simulink model "Sensor"  (R2023b)
settings: Solver=VariableStepAuto  StartTime=0.0  StopTime=10.0  RelTol=1e-3
values from neighbouring files (symbols this model uses):
  a_E_S = 1.495978707e8    (= 149597870.7)    [Sensors.m]
  am2 = 1    [Sensors.m]
  dP = zeros(lenn,lenm)    [Sensors.m]
  Error_horizon = 1.5*pi/180    (= 0.0261799387799)    [Sensors.m]
  Error_mag_HYST = (0.6*60e-6)    (= 3.6e-05)    [Sensors.m]
  Error_mag_ORTHO = deg2rad(0.5)    [Sensors.m]
  Error_sun = 0.5*pi/180    (= 0.00872664625997)    [Sensors.m]
  gnm = Snm.*gnm    [Sensors.m]
  hnm = Snm.*hnm    [Sensors.m]
  i_E = deg2rad(23.45)    [Sensors.m]
  n_E = 2*pi/(365*24*3600)    (= 1.99238499086e-07)    [Sensors.m]
  P = zeros(lenn,lenm)    [Sensors.m]
  R_E = 6371e3    (= 6371000)    [Sensors.m]
  T = 1    [Sensors.m]    (also in sim_with_sensors.m = 2*pi/n)
  w_E = 2*pi/(23*3600+56*60+47)    (= 7.28848621014e-05)    [Sensors.m]
libraries: dspsrcs4 x18, vrlib x2, matrix_library x1, simulink_extras x1
settings Model: Creator=TamimHR  LastModifiedBy=TamimHR

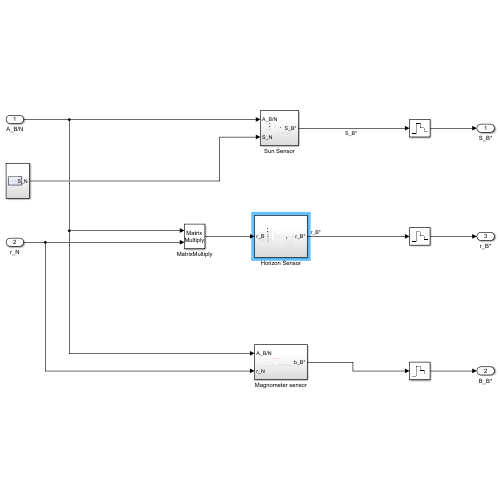
[thumbnail: Simulink's stored preview of the top-level diagram]
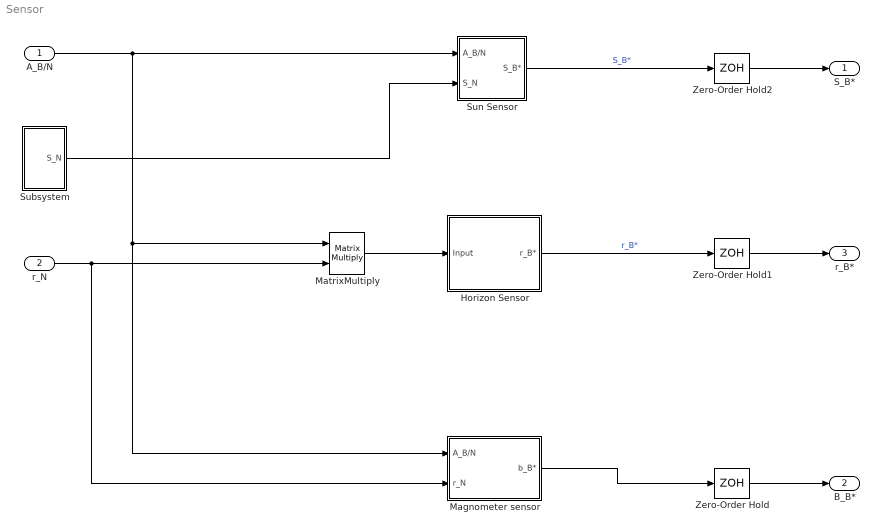
== system Sensor ==
  A_B/N : Inport
  r_N : Inport  Port=2
  Horizon Sensor : Subsystem
  Magnometer sensor : Subsystem
  MatrixMultiply : Product  Multiplication=Matrix(*)
  Subsystem : Subsystem
  Sun Sensor : Subsystem
  Zero-Order Hold : ZeroOrderHold  SampleTime=T
  Zero-Order Hold1 : ZeroOrderHold  SampleTime=T
  Zero-Order Hold2 : ZeroOrderHold  SampleTime=T
  S_B* : Outport
  B_B* : Outport  Port=2
  r_B* : Outport  Port=3
  wires:
  Zero-Order Hold2/1 -> S_B*/1
  A_B/N/1 -> Magnometer sensor/1(A_B/N), MatrixMultiply/1, Sun Sensor/1(A_B/N)
  Sun Sensor/1(S_B*) -> Zero-Order Hold2/1  "S_B*"
  Subsystem/1(S_N) -> Sun Sensor/2(S_N)
  Zero-Order Hold1/1 -> r_B*/1
  Horizon Sensor/1(r_B*) -> Zero-Order Hold1/1  "r_B*"
  r_N/1 -> Magnometer sensor/2(r_N), MatrixMultiply/2
  MatrixMultiply/1 -> Horizon Sensor/1(Input)
  Magnometer sensor/1(b_B*) -> Zero-Order Hold/1
  Zero-Order Hold/1 -> B_B*/1

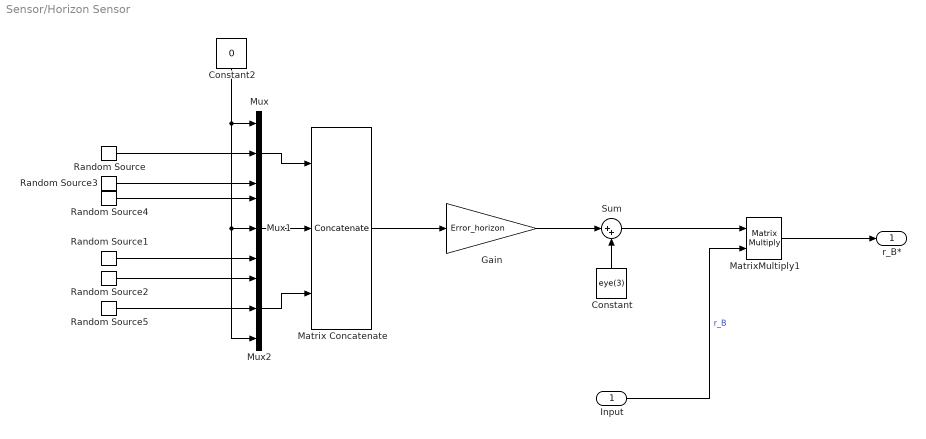
== system Sensor/Horizon Sensor ==
  Input : Inport
  Constant : Constant  Value=eye(3)
  Constant2 : Constant  Value=0
  Gain : Gain  Gain=Error_horizon
  Matrix Concatenate : Concatenate  NumInputs=3  Mode=Multidimensional array  ConcatenateDimension=2
  MatrixMultiply1 : Product  Multiplication=Matrix(*)
  Mux : Mux  Inputs=3
  Mux1 : Mux  Inputs=3
  Mux2 : Mux  Inputs=3
  Random Source : dspsrcs4/Random Source  SrcType=Uniform  NormMethod=Ziggurat  CltLength=12  MinVal=0  MaxVal=1  MeanVal=0  VarVal=1  RepMode=Not repeatable  rawSeed=1  IsInherit=off  SampMode=Discrete  SampTime=1  SampFrame=1  DataType=Double  OutComplex=Real  OutputFrames=off
  Random Source1 : dspsrcs4/Random Source  SrcType=Uniform  NormMethod=Ziggurat  CltLength=12  MinVal=0  MaxVal=1  MeanVal=0  VarVal=1  RepMode=Not repeatable  rawSeed=1  IsInherit=off  SampMode=Discrete  SampTime=1  SampFrame=1  DataType=Double  OutComplex=Real  OutputFrames=off
  Random Source2 : dspsrcs4/Random Source  SrcType=Uniform  NormMethod=Ziggurat  CltLength=12  MinVal=0  MaxVal=1  MeanVal=0  VarVal=1  RepMode=Not repeatable  rawSeed=1  IsInherit=off  SampMode=Discrete  SampTime=1  SampFrame=1  DataType=Double  OutComplex=Real  OutputFrames=off
  Random Source3 : dspsrcs4/Random Source  SrcType=Uniform  NormMethod=Ziggurat  CltLength=12  MinVal=-1  MaxVal=0  MeanVal=0  VarVal=1  RepMode=Not repeatable  rawSeed=1  IsInherit=off  SampMode=Discrete  SampTime=1  SampFrame=1  DataType=Double  OutComplex=Real  OutputFrames=off
  Random Source4 : dspsrcs4/Random Source  SrcType=Uniform  NormMethod=Ziggurat  CltLength=12  MinVal=-1  MaxVal=0  MeanVal=0  VarVal=1  RepMode=Not repeatable  rawSeed=1  IsInherit=off  SampMode=Discrete  SampTime=1  SampFrame=1  DataType=Double  OutComplex=Real  OutputFrames=off
  Random Source5 : dspsrcs4/Random Source  SrcType=Uniform  NormMethod=Ziggurat  CltLength=12  MinVal=-1  MaxVal=0  MeanVal=0  VarVal=1  RepMode=Not repeatable  rawSeed=1  IsInherit=off  SampMode=Discrete  SampTime=1  SampFrame=1  DataType=Double  OutComplex=Real  OutputFrames=off
  Sum : Sum  Inputs=|++
  r_B* : Outport
  wires:
  MatrixMultiply1/1 -> r_B*/1
  Constant2/1 -> Mux/1, Mux1/2, Mux2/3
  Matrix Concatenate/1 -> Gain/1
  Random Source/1 -> Mux/2
  Random Source1/1 -> Mux1/3
  Random Source2/1 -> Mux2/1
  Random Source3/1 -> Mux/3
  Random Source4/1 -> Mux1/1
  Random Source5/1 -> Mux2/2
  Gain/1 -> Sum/1
  Constant/1 -> Sum/2
  Sum/1 -> MatrixMultiply1/1
  Input/1 -> MatrixMultiply1/2  "r_B"
  Mux/1 -> Matrix Concatenate/1
  Mux1/1 -> Matrix Concatenate/2
  Mux2/1 -> Matrix Concatenate/3

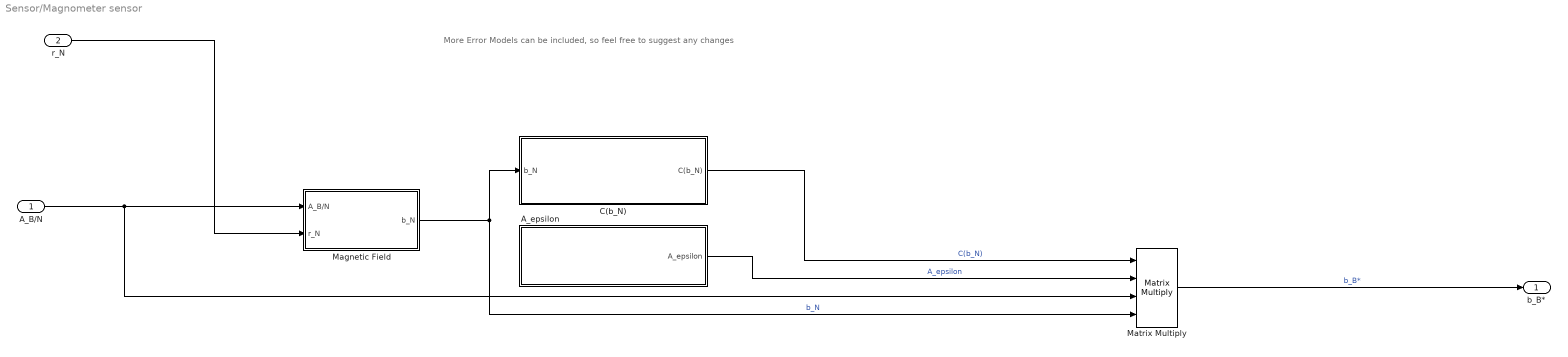
== system Sensor/Magnometer sensor ==
  note: More Error Models can be included, so feel free to suggest any changes
  A_B/N : Inport
  r_N : Inport  Port=2
  A_epsilon : Subsystem
  C(b_N) : Subsystem
  Magnetic Field : Subsystem
  Matrix Multiply : Product  Inputs=4  Multiplication=Matrix(*)
  b_B* : Outport
  wires:
  Matrix Multiply/1 -> b_B*/1  "b_B*"
  A_B/N/1 -> Matrix Multiply/3, Magnetic Field/1(A_B/N)
  Magnetic Field/1(b_N) -> Matrix Multiply/4, C(b_N)/1(b_N)  "b_N"
  A_epsilon/1(A_epsilon) -> Matrix Multiply/2  "A_epsilon"
  C(b_N)/1(C(b_N)) -> Matrix Multiply/1  "C(b_N)"
  r_N/1 -> Magnetic Field/2(r_N)

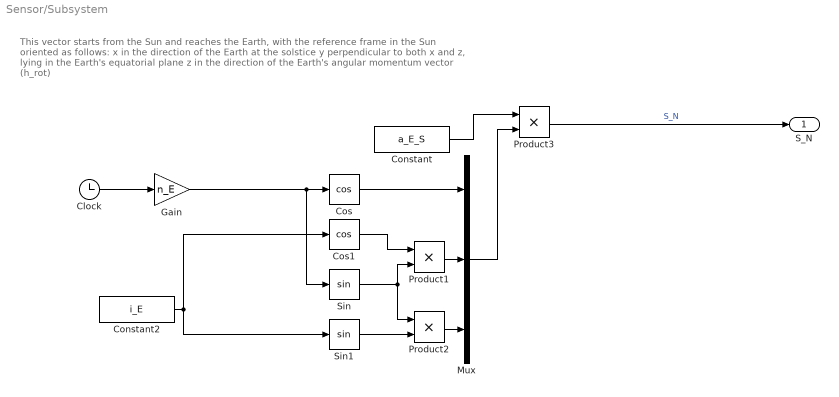
== system Sensor/Subsystem ==
  note: This vector starts from the Sun and reaches the Earth, with the reference frame in the Sun oriented as follows:
      | x in the direction of the Earth at the solstice
      | y perpendicular to both x and z, lying in the Earth's equatorial plane
      | z in the direction of the Earth's angular momentum vector (h_rot)
  Clock : Clock
  Constant : Constant  Value=a_E_S
  Constant2 : Constant  Value=i_E
  Cos : Trigonometry  Operator=cos
  Cos1 : Trigonometry  Operator=cos
  Gain : Gain  Gain=n_E
  Mux : Mux  Inputs=3
  Product1 : Product
  Product2 : Product
  Product3 : Product
  Sin : Trigonometry
  Sin1 : Trigonometry
  S_N : Outport
  wires:
  Gain/1 -> Sin/1, Cos/1
  Clock/1 -> Gain/1
  Mux/1 -> Product3/2
  Sin1/1 -> Product2/2
  Constant/1 -> Product3/1
  Constant2/1 -> Sin1/1, Cos1/1
  Product2/1 -> Mux/3
  Sin/1 -> Product1/2, Product2/1
  Cos1/1 -> Product1/1
  Cos/1 -> Mux/1
  Product1/1 -> Mux/2
  Product3/1 -> S_N/1  "S_N"

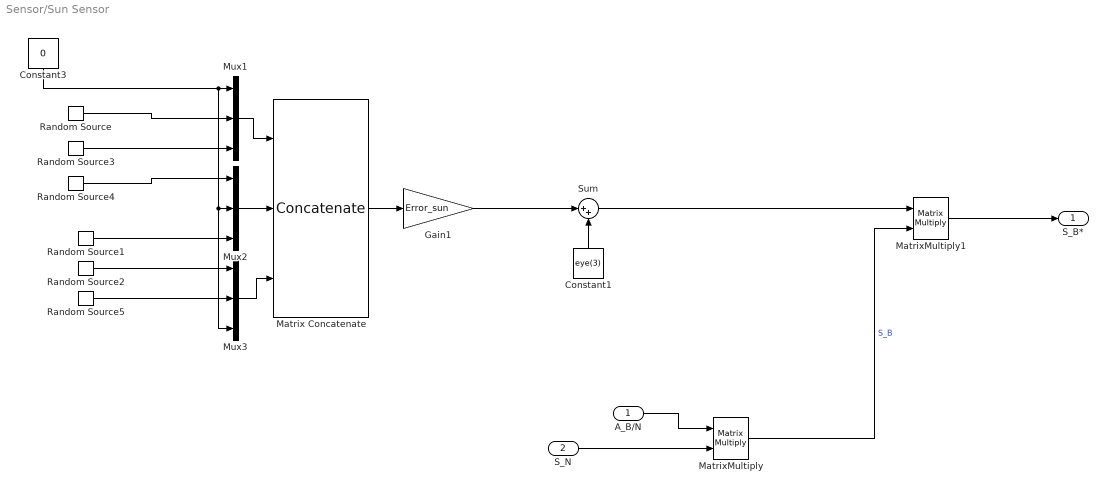
== system Sensor/Sun Sensor ==
  A_B/N : Inport
  S_N : Inport  Port=2
  Constant1 : Constant  Value=eye(3)
  Constant3 : Constant  Value=0
  Gain1 : Gain  Gain=Error_sun
  Matrix Concatenate : Concatenate  NumInputs=3  Mode=Multidimensional array  ConcatenateDimension=2
  MatrixMultiply : Product  Multiplication=Matrix(*)
  MatrixMultiply1 : Product  Multiplication=Matrix(*)
  Mux1 : Mux  Inputs=3
  Mux2 : Mux  Inputs=3
  Mux3 : Mux  Inputs=3
  Random Source : dspsrcs4/Random Source  SrcType=Uniform  NormMethod=Ziggurat  CltLength=12  MinVal=0  MaxVal=1  MeanVal=0  VarVal=1  RepMode=Not repeatable  rawSeed=1  IsInherit=off  SampMode=Discrete  SampTime=1  SampFrame=1  DataType=Double  OutComplex=Real  OutputFrames=off
  Random Source1 : dspsrcs4/Random Source  SrcType=Uniform  NormMethod=Ziggurat  CltLength=12  MinVal=0  MaxVal=1  MeanVal=0  VarVal=1  RepMode=Not repeatable  rawSeed=1  IsInherit=off  SampMode=Discrete  SampTime=1  SampFrame=1  DataType=Double  OutComplex=Real  OutputFrames=off
  Random Source2 : dspsrcs4/Random Source  SrcType=Uniform  NormMethod=Ziggurat  CltLength=12  MinVal=0  MaxVal=1  MeanVal=0  VarVal=1  RepMode=Not repeatable  rawSeed=1  IsInherit=off  SampMode=Discrete  SampTime=1  SampFrame=1  DataType=Double  OutComplex=Real  OutputFrames=off
  Random Source3 : dspsrcs4/Random Source  SrcType=Uniform  NormMethod=Ziggurat  CltLength=12  MinVal=-1  MaxVal=0  MeanVal=0  VarVal=1  RepMode=Not repeatable  rawSeed=1  IsInherit=off  SampMode=Discrete  SampTime=1  SampFrame=1  DataType=Double  OutComplex=Real  OutputFrames=off
  Random Source4 : dspsrcs4/Random Source  SrcType=Uniform  NormMethod=Ziggurat  CltLength=12  MinVal=-1  MaxVal=0  MeanVal=0  VarVal=1  RepMode=Not repeatable  rawSeed=1  IsInherit=off  SampMode=Discrete  SampTime=1  SampFrame=1  DataType=Double  OutComplex=Real  OutputFrames=off
  Random Source5 : dspsrcs4/Random Source  SrcType=Uniform  NormMethod=Ziggurat  CltLength=12  MinVal=-1  MaxVal=0  MeanVal=0  VarVal=1  RepMode=Not repeatable  rawSeed=1  IsInherit=off  SampMode=Discrete  SampTime=1  SampFrame=1  DataType=Double  OutComplex=Real  OutputFrames=off
  Sum : Sum  Inputs=|++
  S_B* : Outport
  wires:
  Constant3/1 -> Mux2/2, Mux3/3, Mux1/1
  Sum/1 -> MatrixMultiply1/1
  Random Source2/1 -> Mux3/1
  Random Source4/1 -> Mux2/1
  Constant1/1 -> Sum/2
  MatrixMultiply/1 -> MatrixMultiply1/2  "S_B"
  A_B/N/1 -> MatrixMultiply/1
  MatrixMultiply1/1 -> S_B*/1
  Mux3/1 -> Matrix Concatenate/3
  Mux2/1 -> Matrix Concatenate/2
  Mux1/1 -> Matrix Concatenate/1
  Random Source5/1 -> Mux3/2
  Random Source/1 -> Mux1/2
  Gain1/1 -> Sum/1
  Random Source1/1 -> Mux2/3
  Random Source3/1 -> Mux1/3
  Matrix Concatenate/1 -> Gain1/1
  S_N/1 -> MatrixMultiply/2

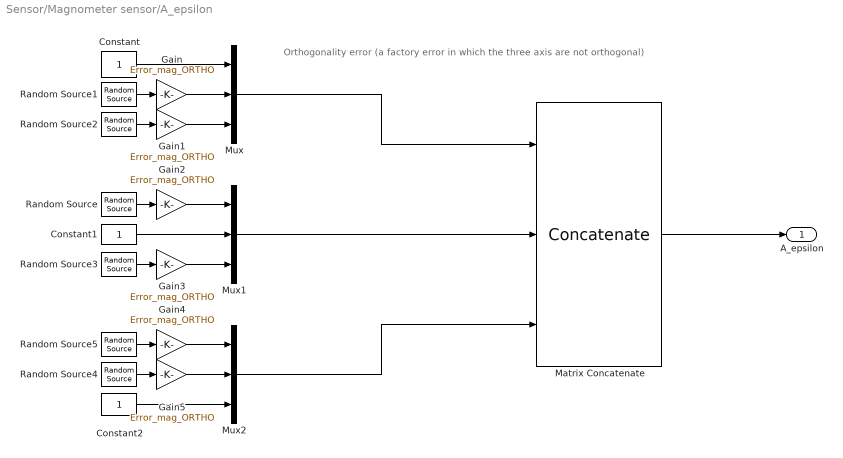
== system Sensor/Magnometer sensor/A_epsilon ==
  note: Orthogonality error (a factory error in which the three axis are not orthogonal)
  Constant : Constant
  Constant1 : Constant
  Constant2 : Constant
  Gain{,1..5} (6 alike) : Gain  Gain=Error_mag_ORTHO
  Matrix Concatenate : Concatenate  NumInputs=3  Mode=Multidimensional array  ConcatenateDimension=2
  Mux : Mux  Inputs=3
  Mux1 : Mux  Inputs=3
  Mux2 : Mux  Inputs=3
  Random Source{,1..5} (6 alike) : dspsrcs4/Random Source  SrcType=Uniform  NormMethod=Ziggurat  CltLength=12  MinVal=-1  MaxVal=1  MeanVal=0  VarVal=25  RepMode=Not repeatable  rawSeed=1  IsInherit=off  SampMode=Continuous  SampTime=1  SampFrame=1  DataType=Double  OutComplex=Real  OutputFrames=off
  A_epsilon : Outport
  wires:
  Random Source4/1 -> Gain5/1
  Constant/1 -> Mux/1
  Mux/1 -> Matrix Concatenate/1
  Random Source1/1 -> Gain/1
  Random Source/1 -> Gain2/1
  Mux1/1 -> Matrix Concatenate/2
  Random Source2/1 -> Gain1/1
  Random Source3/1 -> Gain3/1
  Random Source5/1 -> Gain4/1
  Mux2/1 -> Matrix Concatenate/3
  Matrix Concatenate/1 -> A_epsilon/1
  Gain/1 -> Mux/2
  Gain1/1 -> Mux/3
  Gain2/1 -> Mux1/1
  Gain3/1 -> Mux1/3
  Gain4/1 -> Mux2/1
  Gain5/1 -> Mux2/2
  Constant1/1 -> Mux1/2
  Constant2/1 -> Mux2/3

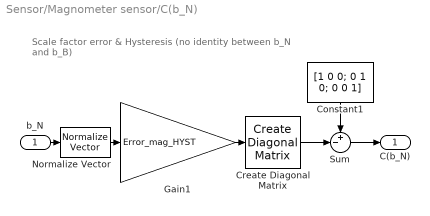
== system Sensor/Magnometer sensor/C(b_N) ==
  note: Scale factor error & Hysteresis (no identity between b_N and b_B)
  b_N : Inport
  Constant1 : Constant  Value=[1 0 0; 0 1 0; 0 0 1]
  Create Diagonal Matrix : matrix_library/Create Diagonal Matrix
      settings: LibrarySourceBlock=|
      | simulink/Matrix
      | Operations/Create Diagonal
      | Matrix
  Gain1 : Gain  Gain=Error_mag_HYST
  Normalize Vector : vrlib/Utilities/Normalize Vector  maxzero=0
  Sum : Sum  Inputs=+-|
  C(b_N) : Outport
  wires:
  Normalize Vector/1 -> Gain1/1
  Gain1/1 -> Create Diagonal Matrix/1
  Constant1/1 -> Sum/1
  Sum/1 -> C(b_N)/1
  b_N/1 -> Normalize Vector/1
  Create Diagonal Matrix/1 -> Sum/2

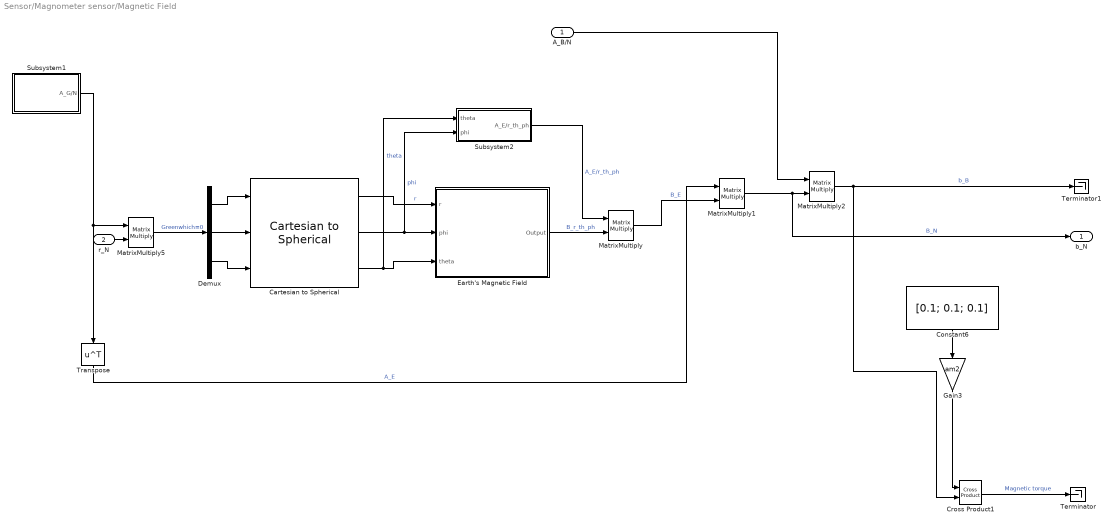
== system Sensor/Magnometer sensor/Magnetic Field ==
  A_B/N : Inport
  r_N : Inport  Port=2
  Cartesian to Spherical : simulink_extras/Transformations/Cartesian to Spherical
  Constant6 : Constant  Value=[0.1; 0.1; 0.1]
  Cross Product1 : vrlib/Utilities/Cross Product
  Demux : Demux  Outputs=3
  Earth's Magnetic Field : Subsystem
  Gain3 : Gain  Gain=am2
  MatrixMultiply{,1..2,5} (4 alike) : Product  Multiplication=Matrix(*)
  Subsystem1 : Subsystem
  Subsystem2 : Subsystem
  Terminator : Terminator
  Terminator1 : Terminator
  Transpose : Math  Operator=transpose
  b_N : Outport
  wires:
  Demux/3 -> Cartesian to Spherical/3
  Subsystem2/1(A_E/r_th_ph) -> MatrixMultiply/1  "A_E/r_th_ph"
  MatrixMultiply1/1 -> b_N/1, MatrixMultiply2/2  "B_N"
  Gain3/1 -> Cross Product1/1
  Cartesian to Spherical/3 -> Subsystem2/1(theta), Earth's Magnetic Field/3(theta)  "theta"
  MatrixMultiply/1 -> MatrixMultiply1/2  "B_E"
  Earth's Magnetic Field/1(Output) -> MatrixMultiply/2  "B_r_th_ph"
  Constant6/1 -> Gain3/1
  MatrixMultiply2/1 -> Terminator1/1, Cross Product1/2  "b_B"
  Transpose/1 -> MatrixMultiply1/1  "A_E"
  A_B/N/1 -> MatrixMultiply2/1
  Cross Product1/1 -> Terminator/1  "Magnetic torque"
  Cartesian to Spherical/2 -> Subsystem2/2(phi), Earth's Magnetic Field/2(phi)  "phi"
  Cartesian to Spherical/1 -> Earth's Magnetic Field/1(r)  "r"
  Demux/2 -> Cartesian to Spherical/2
  MatrixMultiply5/1 -> Demux/1  "Greenwhich=0"
  Subsystem1/1(A_G/N) -> MatrixMultiply5/1, Transpose/1
  Demux/1 -> Cartesian to Spherical/1
  r_N/1 -> MatrixMultiply5/2

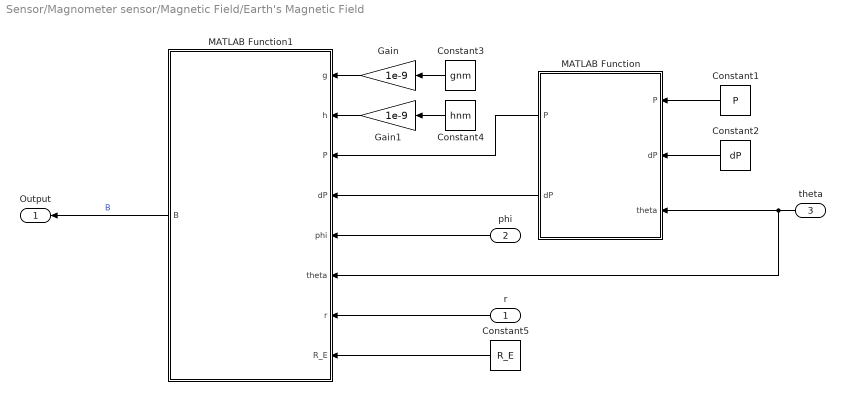
== system Sensor/Magnometer sensor/Magnetic Field/Earth's Magnetic Field ==
  r : Inport
  phi : Inport  Port=2
  theta : Inport  Port=3
  Constant1 : Constant  Value=P
  Constant2 : Constant  Value=dP
  Constant3 : Constant  Value=gnm
  Constant4 : Constant  Value=hnm
  Constant5 : Constant  Value=R_E
  Gain : Gain  Gain=1e-9
  Gain1 : Gain  Gain=1e-9
  MATLAB Function : MATLAB Function  TreatAsAtomicUnit=on
  MATLAB Function1 : MATLAB Function  TreatAsAtomicUnit=on
  Output : Outport
  wires:
  Constant1/1 -> MATLAB Function/1("P ")
  Constant2/1 -> MATLAB Function/2("dP ")
  theta/1 -> MATLAB Function/3(theta), MATLAB Function1/6(theta)
  Constant3/1 -> Gain/1
  Constant4/1 -> Gain1/1
  phi/1 -> MATLAB Function1/5(phi)
  r/1 -> MATLAB Function1/7(r)
  Constant5/1 -> MATLAB Function1/8(R_E)
  MATLAB Function1/1(B) -> Output/1  "B"
  MATLAB Function/1(P) -> MATLAB Function1/3(P)
  MATLAB Function/2(dP) -> MATLAB Function1/4(dP)
  Gain/1 -> MATLAB Function1/1(g)
  Gain1/1 -> MATLAB Function1/2(h)

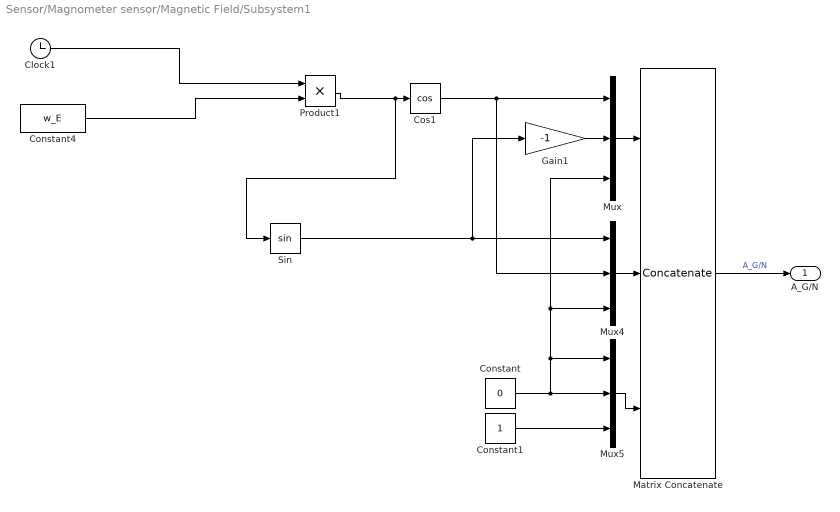
== system Sensor/Magnometer sensor/Magnetic Field/Subsystem1 ==
  Clock1 : Clock
  Constant : Constant  Value=0
  Constant1 : Constant
  Constant4 : Constant  Value=w_E
  Cos1 : Trigonometry  Operator=cos
  Gain1 : Gain  Gain=-1
  Matrix Concatenate : Concatenate  NumInputs=3  Mode=Multidimensional array  ConcatenateDimension=2
  Mux : Mux  Inputs=3
  Mux4 : Mux  Inputs=3
  Mux5 : Mux  Inputs=3
  Product1 : Product
  Sin : Trigonometry
  A_G/N : Outport
  wires:
  Mux/1 -> Matrix Concatenate/1
  Matrix Concatenate/1 -> A_G/N/1  "A_G/N"
  Constant1/1 -> Mux5/3
  Cos1/1 -> Mux/1, Mux4/2
  Gain1/1 -> Mux/2
  Constant/1 -> Mux/3, Mux4/3, Mux5/1, Mux5/2
  Mux4/1 -> Matrix Concatenate/2
  Sin/1 -> Mux4/1, Gain1/1
  Mux5/1 -> Matrix Concatenate/3
  Product1/1 -> Sin/1, Cos1/1
  Constant4/1 -> Product1/2
  Clock1/1 -> Product1/1

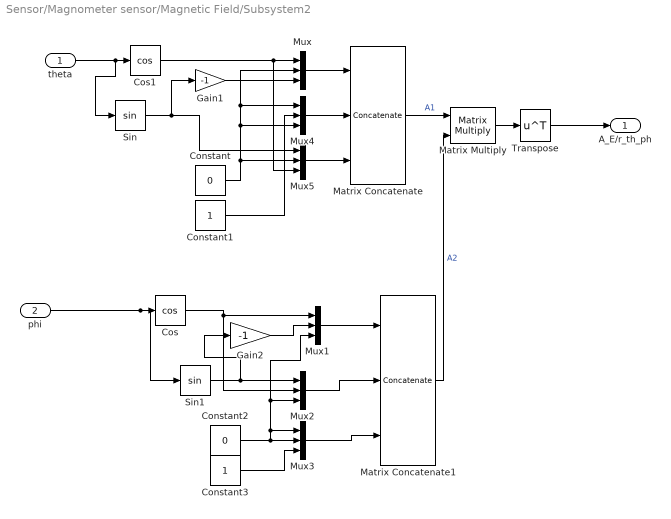
== system Sensor/Magnometer sensor/Magnetic Field/Subsystem2 ==
  theta : Inport
  phi : Inport  Port=2
  Constant : Constant  Value=0
  Constant1 : Constant
  Constant2 : Constant  Value=0
  Constant3 : Constant
  Cos : Trigonometry  Operator=cos
  Cos1 : Trigonometry  Operator=cos
  Gain1 : Gain  Gain=-1
  Gain2 : Gain  Gain=-1
  Matrix Concatenate : Concatenate  NumInputs=3  Mode=Multidimensional array  ConcatenateDimension=2
  Matrix Concatenate1 : Concatenate  NumInputs=3  Mode=Multidimensional array  ConcatenateDimension=2
  Matrix Multiply : Product  Multiplication=Matrix(*)
  Mux{,1..5} (6 alike) : Mux  Inputs=3
  Sin : Trigonometry
  Sin1 : Trigonometry
  Transpose : Math  Operator=transpose
  A_E/r_th_ph : Outport
  wires:
  Mux/1 -> Matrix Concatenate/1
  Mux4/1 -> Matrix Concatenate/2
  Mux5/1 -> Matrix Concatenate/3
  Mux1/1 -> Matrix Concatenate1/1
  Mux2/1 -> Matrix Concatenate1/2
  Mux3/1 -> Matrix Concatenate1/3
  Matrix Multiply/1 -> Transpose/1
  phi/1 -> Sin1/1, Cos/1
  theta/1 -> Sin/1, Cos1/1
  Cos1/1 -> Mux5/3, Mux/1
  Sin1/1 -> Mux2/1, Gain2/1
  Sin/1 -> Mux5/1, Gain1/1
  Constant/1 -> Mux/2, Mux4/1, Mux4/3, Mux5/2
  Gain1/1 -> Mux/3
  Constant1/1 -> Mux4/2
  Matrix Concatenate/1 -> Matrix Multiply/1  "A1"
  Matrix Concatenate1/1 -> Matrix Multiply/2  "A2"
  Cos/1 -> Mux2/2, Mux1/1
  Gain2/1 -> Mux1/2
  Constant2/1 -> Mux2/3, Mux1/3, Mux3/1, Mux3/2
  Constant3/1 -> Mux3/3
  Transpose/1 -> A_E/r_th_ph/1

== matlab function Sensor/Magnometer sensor/Magnetic Field/Earth's Magnetic Field/MATLAB Function ==
  data: P input; P output size=lenm; dP input; theta input; dP output size=lenm
function [P, dP] = CalculateP(P,dP,theta)
lenn = length(P(:,1));
P00 = 1;
P(1,1) = cos(theta)*P00;
dP(1,1) = -sin(theta)*P00;
n=2;
m=1;
K= ((n-1)^2-m^2)/((2*n-1)*(2*n-3));
P(2,1) = cos(theta)*P(1,1)-K*P00;
dP(2,1) = -sin(theta)*P(1,1);

n = 0;
m = 0;
for j = 3:lenn
    n = n+1;
    K= ((n-1)^2-m^2)/((2*n-1)*(2*n-3));
    P(j,1) = cos(theta)*P(j-1,1)-K*P(j-2,1);
    dP(j,1) = -sin(theta)*P(j-1,1);
end 

P(1,2) = sin(theta)*P00;
dP(1,2) = cos(theta)*P00;

n =1;
m = 0;
k=3;
for j=2:lenn
    n = 1+n;
    for i=2:k
        m = m+1;
        K= ((n-1)^2-m^2)/((2*n-1)*(2*n-3));
        if m == n
            P(j,i) = sin(theta)*P(j-1,j-1);
            dP(j,i) = cos(theta)*P(j-1,j-1);
        elseif K == 0
            P(j,i) = cos(theta)*P(j-1,i);
            dP(j,i) = -sin(theta)*P(j-1,i);
        else
            P(j,i) = cos(theta)*P(j-1,i)-K*P(j-2,i);
            dP(j,i) = -sin(theta)*P(j-1,i)-K*P(j-2,i);
        end

    end
    m=0;
    k = k+1;
end
end

== matlab function Sensor/Magnometer sensor/Magnetic Field/Earth's Magnetic Field/MATLAB Function1 ==
  data: g input; B output; h input; P input; dP input; phi input; theta input; r input; R_E input
function B = MagneticField(g,h,P,dP,phi,theta,r,R_E)
k = length(g(:,1));
Br = 0;
Btheta = 0;
Bphi = 0;

for n = 1:k
    m = 0;
    for i=1:n
        
        Br = Br + (R_E/r)^(n+2)*(n+1)*( g(n,i)*cos(m*phi) + h(n,i)*sin(m*phi) )*P(n,i);
        Btheta = Btheta - (R_E/r)^(n+2)*( g(n,i)*cos(m*phi) + h(n,i)*sin(m*phi) )*dP(n,i);
        Bphi = Bphi -1/sin(theta)*(R_E/r)^(n+2)*m*(-g(n,i)*sin(m*phi) + h(n,i)*cos(m*phi))*P(n,i);
        
        m = m+1;
    end
end

B = [Btheta Bphi Br]';

end
